simulink library "lib_inverse_park_transform"  (R2023a)
settings: Solver=VariableStepAuto  StartTime=0.0  StopTime=10.0  RelTol=1e-3
libraries: vhit_control_library x2
settings Model: Creator=cav2ofo  LastModifiedBy=lenovo
settings OptimizationCC: ReuseModelBlockBuffer=off

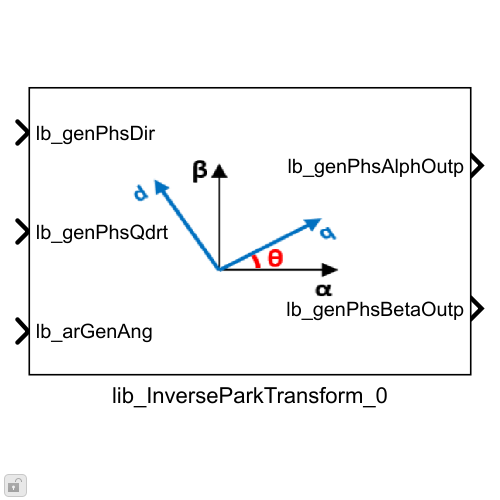
[thumbnail: Simulink's stored preview of the top-level diagram]
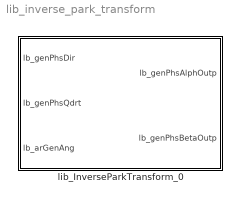
== system lib_inverse_park_transform ==
  lib_InverseParkTransform_0 : Subsystem  VariantControl=ClarkTransf_MIL_flo  mask{lb_parSelRotFrmeAxis=d-axis}
      mask prompts: lb_parSelRotFrmeAxis "Select an axis align:"
      mask TypeOptions lb_parSelRotFrmeAxis: d-axis | q-axis
      mask DialogControl DescGroupVar Prompt: Park Transform
      mask DialogControl DescTextVar Prompt: VHIT Control Library
      mask DialogControl clarkeDesc Prompt: This block performs Inverse Park transformation on rotating reference frame (d-q) inputs into stationary reference frame (alpha-beta) output.
      mask DialogControl blockParam Prompt: Block Parameters
      mask DialogControl Control2 Prompt: By default aligns d-axis with alpha-axis. Select q-axis from the following list.
      mask Display: image('ParkTransf.PNG'); % Use "Edit Image" on toolstrip to change.

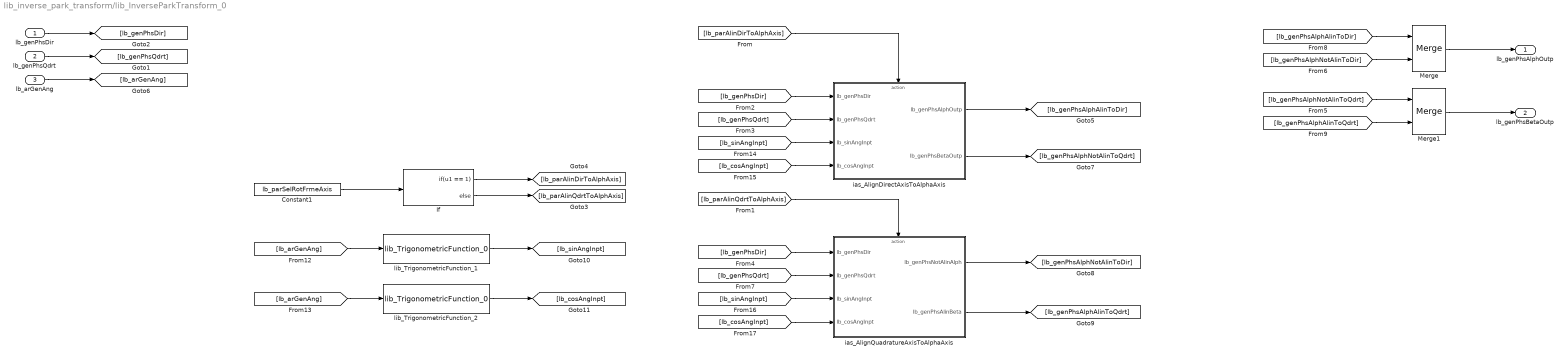
== system lib_inverse_park_transform/lib_InverseParkTransform_0 ==
  lb_genPhsDir : Inport
  lb_genPhsQdrt : Inport  Port=2
  lb_arGenAng : Inport  Port=3
  Constant1 : Constant  Value=lb_parSelRotFrmeAxis  OutDataTypeStr=int8
  If : If  IfExpression=u1 == 1
  Merge : Merge
  Merge1 : Merge
  ias_AlignDirectAxisToAlphaAxis : Subsystem  TreatAsAtomicUnit=on
  ias_AlignQuadratureAxisToAlphaAxis : Subsystem  TreatAsAtomicUnit=on
  lib_TrigonometricFunction_1 : vhit_control_library/lib_TrigonometricFunction_0  lb_parSelSigType=Sine  lb_parLktSizeStr=1024  lb_parOutpDataType=fixdt(1,16,2^-14,0)
  lib_TrigonometricFunction_2 : vhit_control_library/lib_TrigonometricFunction_0  lb_parSelSigType=Cosine  lb_parLktSizeStr=1024  lb_parOutpDataType=fixdt(1,16,2^-14,0)
  lb_genPhsAlphOutp : Outport  VectorParamsAs1DForOutWhenUnconnected=off
  lb_genPhsBetaOutp : Outport  Port=2  VectorParamsAs1DForOutWhenUnconnected=off
  wires:
  lb_arGenAng/1 -> [lb_arGenAng]
  lb_genPhsQdrt/1 -> [lb_genPhsQdrt]
  lb_genPhsDir/1 -> [lb_genPhsDir]
  Constant1/1 -> If/1
  [lb_parAlinDirToAlphAxis] -> ias_AlignDirectAxisToAlphaAxis/Action
  [lb_parAlinQdrtToAlphAxis] -> ias_AlignQuadratureAxisToAlphaAxis/Action
  [lb_genPhsDir] -> ias_AlignDirectAxisToAlphaAxis/1(lb_genPhsDir)
  [lb_genPhsQdrt] -> ias_AlignDirectAxisToAlphaAxis/2(lb_genPhsQdrt)
  [lb_genPhsDir] -> ias_AlignQuadratureAxisToAlphaAxis/1(lb_genPhsDir)
  [lb_genPhsQdrt] -> ias_AlignQuadratureAxisToAlphaAxis/2(lb_genPhsQdrt)
  ias_AlignDirectAxisToAlphaAxis/1(lb_genPhsAlphOutp) -> [lb_genPhsAlphAlinToDir]
  ias_AlignDirectAxisToAlphaAxis/2(lb_genPhsBetaOutp) -> [lb_genPhsAlphNotAlinToQdrt]
  ias_AlignQuadratureAxisToAlphaAxis/1(lb_genPhsNotAlinAlph) -> [lb_genPhsAlphNotAlinToDir]
  ias_AlignQuadratureAxisToAlphaAxis/2(lb_genPhsAlinBeta) -> [lb_genPhsAlphAlinToQdrt]
  [lb_genPhsAlphAlinToDir] -> Merge/1
  [lb_genPhsAlphNotAlinToDir] -> Merge/2
  [lb_genPhsAlphAlinToQdrt] -> Merge1/2
  [lb_genPhsAlphNotAlinToQdrt] -> Merge1/1
  If/2 -> [lb_parAlinQdrtToAlphAxis]
  If/1 -> [lb_parAlinDirToAlphAxis]
  Merge1/1 -> lb_genPhsBetaOutp/1
  Merge/1 -> lb_genPhsAlphOutp/1
  [lb_arGenAng] -> lib_TrigonometricFunction_2/1
  [lb_arGenAng] -> lib_TrigonometricFunction_1/1
  lib_TrigonometricFunction_2/1 -> [lb_cosAngInpt]
  lib_TrigonometricFunction_1/1 -> [lb_sinAngInpt]
  [lb_sinAngInpt] -> ias_AlignDirectAxisToAlphaAxis/3(lb_sinAngInpt)
  [lb_cosAngInpt] -> ias_AlignDirectAxisToAlphaAxis/4(lb_cosAngInpt)
  [lb_sinAngInpt] -> ias_AlignQuadratureAxisToAlphaAxis/3(lb_sinAngInpt)
  [lb_cosAngInpt] -> ias_AlignQuadratureAxisToAlphaAxis/4(lb_cosAngInpt)

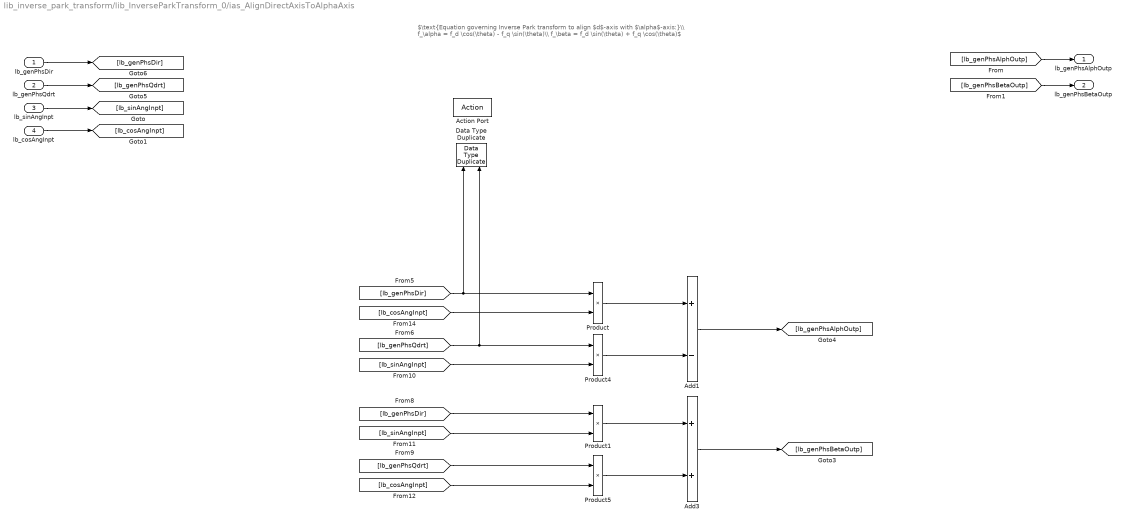
== system lib_inverse_park_transform/lib_InverseParkTransform_0/ias_AlignDirectAxisToAlphaAxis ==
  note: $\text{Equation governing Inverse Park transform to align $d$-axis with $\alpha$-axis:}\\ f_\alpha = f_d \cos(\theta) - f_q \sin(\theta)\\ f_\beta = f_d \sin(\theta) + f_q \cos(\theta)$
  lb_genPhsDir : Inport
  lb_genPhsQdrt : Inport  Port=2
  lb_sinAngInpt : Inport  Port=3
  lb_cosAngInpt : Inport  Port=4
  Action Port : ActionPort
  Add1 : Sum  Inputs=+-  OutDataTypeStr=Inherit: Same as first input
  Add3 : Sum  OutDataTypeStr=Inherit: Same as first input
  Data Type Duplicate : DataTypeDuplicate
  Product{,1,4..5} (4 alike) : Product  OutDataTypeStr=Inherit: Same as first input
  lb_genPhsAlphOutp : Outport  VectorParamsAs1DForOutWhenUnconnected=off
  lb_genPhsBetaOutp : Outport  Port=2  VectorParamsAs1DForOutWhenUnconnected=off
  wires:
  [lb_genPhsAlphOutp] -> lb_genPhsAlphOutp/1
  [lb_genPhsBetaOutp] -> lb_genPhsBetaOutp/1
  [lb_genPhsDir] -> Data Type Duplicate/1, Product/1
  [lb_cosAngInpt] -> Product/2
  Add1/1 -> [lb_genPhsAlphOutp]
  Product/1 -> Add1/1
  [lb_genPhsQdrt] -> Product4/1, Data Type Duplicate/2
  Product4/1 -> Add1/2
  lb_genPhsQdrt/1 -> [lb_genPhsQdrt]
  lb_genPhsDir/1 -> [lb_genPhsDir]
  [lb_sinAngInpt] -> Product4/2
  [lb_sinAngInpt] -> Product1/2
  Product1/1 -> Add3/1
  Add3/1 -> [lb_genPhsBetaOutp]
  [lb_cosAngInpt] -> Product5/2
  [lb_genPhsDir] -> Product1/1
  Product5/1 -> Add3/2
  [lb_genPhsQdrt] -> Product5/1
  lb_cosAngInpt/1 -> [lb_cosAngInpt]
  lb_sinAngInpt/1 -> [lb_sinAngInpt]

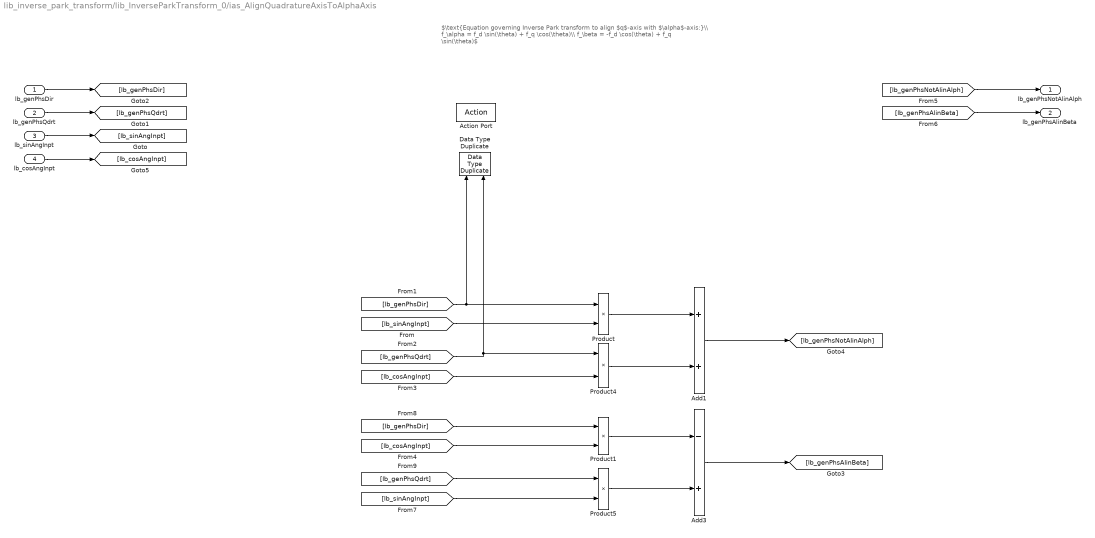
== system lib_inverse_park_transform/lib_InverseParkTransform_0/ias_AlignQuadratureAxisToAlphaAxis ==
  note: $\text{Equation governing Inverse Park transform to align $q$-axis with $\alpha$-axis:}\\ f_\alpha = f_d \sin(\theta) + f_q \cos(\theta)\\ f_\beta = -f_d \cos(\theta) + f_q \sin(\theta)$
  lb_genPhsDir : Inport
  lb_genPhsQdrt : Inport  Port=2
  lb_sinAngInpt : Inport  Port=3
  lb_cosAngInpt : Inport  Port=4
  Action Port : ActionPort
  Add1 : Sum  OutDataTypeStr=Inherit: Same as first input
  Add3 : Sum  Inputs=-+  OutDataTypeStr=Inherit: Same as first input
  Data Type Duplicate : DataTypeDuplicate
  Product{,1,4..5} (4 alike) : Product  OutDataTypeStr=Inherit: Same as first input
  lb_genPhsNotAlinAlph : Outport  VectorParamsAs1DForOutWhenUnconnected=off
  lb_genPhsAlinBeta : Outport  Port=2  VectorParamsAs1DForOutWhenUnconnected=off
  wires:
  lb_genPhsQdrt/1 -> [lb_genPhsQdrt]
  lb_genPhsDir/1 -> [lb_genPhsDir]
  [lb_genPhsNotAlinAlph] -> lb_genPhsNotAlinAlph/1
  [lb_genPhsAlinBeta] -> lb_genPhsAlinBeta/1
  Product4/1 -> Add1/2
  [lb_genPhsDir] -> Data Type Duplicate/1, Product/1
  [lb_sinAngInpt] -> Product/2
  Product/1 -> Add1/1
  Add1/1 -> [lb_genPhsNotAlinAlph]
  [lb_sinAngInpt] -> Product5/2
  [lb_genPhsQdrt] -> Product5/1
  Product1/1 -> Add3/1
  [lb_genPhsDir] -> Product1/1
  [lb_cosAngInpt] -> Product4/2
  Product5/1 -> Add3/2
  Add3/1 -> [lb_genPhsAlinBeta]
  [lb_genPhsQdrt] -> Data Type Duplicate/2, Product4/1
  [lb_cosAngInpt] -> Product1/2
  lb_sinAngInpt/1 -> [lb_sinAngInpt]
  lb_cosAngInpt/1 -> [lb_cosAngInpt]
